simulink model "Asservissement_Robot"  (R2019b)
settings: Solver=VariableStepAuto  StartTime=0.0  StopTime=10.0  RelTol=1e-3
undefined symbols (not defined in the file): Cr, f, J, K, Ke, Km, R
libraries: simulink x1
settings Model: Creator=Shanly  LastModifiedBy=noecl

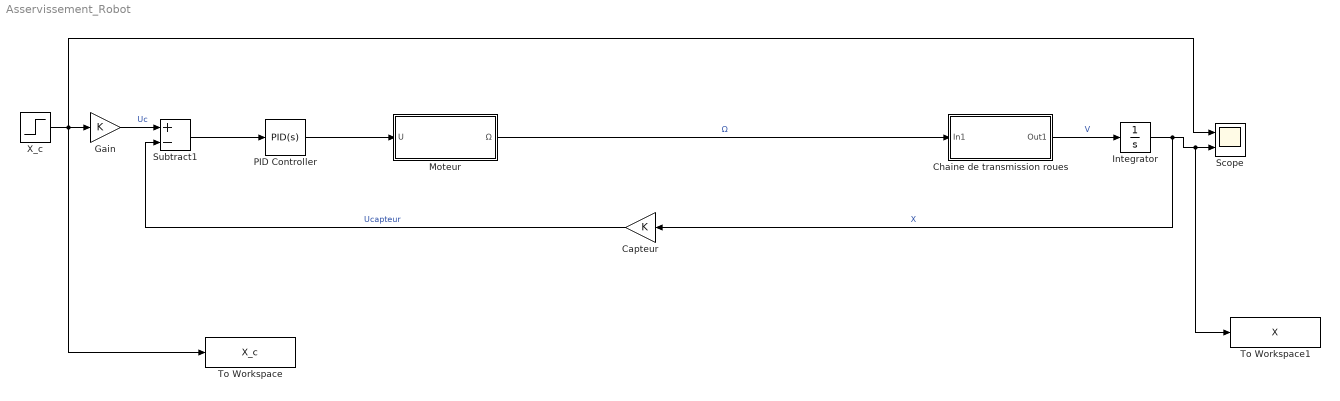
== system Asservissement_Robot ==
  "Capteur " : Gain  Gain=K
  Chaine de transmission roues : Subsystem
  Gain : Gain  Gain=K
  Integrator : Integrator
  "Moteur " : Subsystem
  PID Controller : simulink/Continuous/PID Controller  Controller=PID  Form=Parallel  TimeDomain=Continuous-time  SampleTime=-1  IntegratorMethod=Forward Euler  FilterMethod=Forward Euler  ControllerParametersSource=internal  P=29.7041706933747  I=53.4908346202361  D=2.48390648241735  UseFilter=on  N=28847.9278775678  TunerSelectOption=Transfer Function Based (PID Tuner App)  InitialConditionSource=internal  InitialConditionForIntegrator=0  InitialConditionForFilter=0  DifferentiatorICPrevScaledInput=0  ExternalReset=none  TrackingMode=off  Kt=1  LimitOutput=off  UpperSaturationLimit=inf  LowerSaturationLimit=-inf  LinearizeAsGain=on  AntiWindupMode=none  Kb=1  POutMin=[]  POutMax=[]  IOutMin=[]  IOutMax=[]  DOutMin=[]  DOutMax=[]  NOutMin=[]  NOutMax=[]  SumOutMin=[]  SumOutMax=[]  SaturationOutMin=[]  SaturationOutMax=[]  PParamMin=[]  PParamMax=[]  IParamMin=[]  IParamMax=[]  DParamMin=[]  DParamMax=[]  NParamMin=[]  NParamMax=[]  KbParamMin=[]  KbParamMax=[]  KtParamMin=[]  KtParamMax=[]  KbOutMin=[]  KbOutMax=[]  KtOutMin=[]  KtOutMax=[]  IntegratorOutMin=[]  IntegratorOutMax=[]  FilterOutMin=[]  FilterOutMax=[]  SumI1OutMin=[]  SumI1OutMax=[]  SumI2OutMin=[]  SumI2OutMax=[]  SumI3OutMin=[]  SumI3OutMax=[]  SumI4OutMin=[]  SumI4OutMax=[]  SumDOutMin=[]  SumDOutMax=[]  DifferentiatorOutMin=[]  DifferentiatorOutMax=[]  FilterDiffOutCoefMin=[]  FilterDiffOutCoefMax=[]  ReciprocalOutMin=[]  ReciprocalOutMax=[]  SumDenOutMin=[]  SumDenOutMax=[]  SumNumOutMin=[]  SumNumOutMax=[]  DivideOutMin=[]  DivideOutMax=[]  IntegratorContinuousStateAttributes=''  IntegratorStateMustResolveToSignalObject=off  IntegratorRTWStateStorageClass=Auto  FilterContinuousStateAttributes=''  FilterStateMustResolveToSignalObject=off  FilterRTWStateStorageClass=Auto  ParallelPVariant=InternalParameters  IdealPVariant=Disabled  IVariant=InternalParameters  DVariant=InternalParameters  IntegratorVariant=Continuous  SatVariant=Disabled  AWVariant=Passthrough  PCopyVariant=Disabled  TRVariant=Disabled  FdbkBlocksVariant=Forward  IdealPFdbkVariant=Disabled  SatFdbkVariant=Disabled  DerivativeFilterVariant=ContFilter  NVariant=InternalParameters  NCopyVariant=Disabled  FilterICVariant=InternalICsFilter  IntegratorICVariant=InternalICs  ExternalResetVariant=Disabled  TRSumVariant=Passthrough  SumFdbkVariant=Disabled  SumVariant=Sum_PID
  Scope : Scope  NumInputPorts=2
  Subtract1 : Sum  Inputs=+-
  To Workspace : ToWorkspace  VariableName=X_c  SaveFormat=Timeseries  SampleTime=-1
  To Workspace1 : ToWorkspace  VariableName=X  SaveFormat=Timeseries  SampleTime=-1
  X_c : Step  SampleTime=0
  wires:
  "Moteur "/1(Ω) -> Chaine de transmission roues/1(In1)  "Ω"
  PID Controller/1 -> "Moteur "/1(U)
  Chaine de transmission roues/1(Out1) -> Integrator/1  "V"
  Integrator/1 -> "Capteur "/1, To Workspace1/1, Scope/2  "X"
  X_c/1 -> To Workspace/1, Gain/1, Scope/1
  Subtract1/1 -> PID Controller/1
  "Capteur "/1 -> Subtract1/2  "Ucapteur"
  Gain/1 -> Subtract1/1  "Uc"

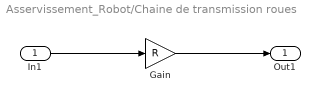
== system Asservissement_Robot/Chaine de transmission roues ==
  In1 : Inport
  Gain : Gain  Gain=R
  Out1 : Outport
  wires:
  In1/1 -> Gain/1
  Gain/1 -> Out1/1

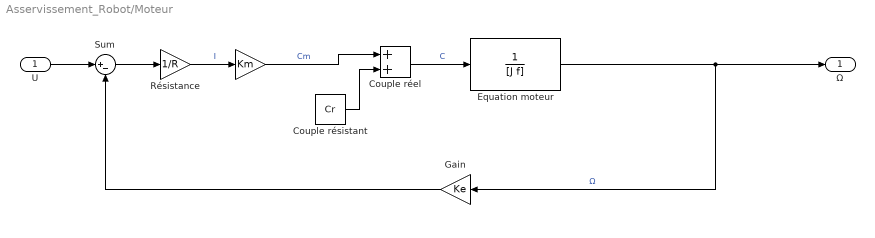
== system Asservissement_Robot/Moteur  ==
  U : Inport
  " " : Gain  Gain=Km
  Couple réel : Sum
  Couple résistant : Constant  Value=Cr
  Equation moteur : TransferFcn  Denominator=[J f]
  Gain : Gain  Gain=Ke
  Résistance : Gain  Gain=1/R
  Sum : Sum  Inputs=|+-
  Ω : Outport
  wires:
  U/1 -> Sum/1
  Equation moteur/1 -> Gain/1, Ω/1  "Ω"
  Résistance/1 -> " "/1  "I"
  " "/1 -> Couple réel/1  "Cm"
  Couple réel/1 -> Equation moteur/1  "C"
  Couple résistant/1 -> Couple réel/2
  Sum/1 -> Résistance/1
  Gain/1 -> Sum/2
